simulink model "VerificaLQR"  (R2025b)
settings: Solver=VariableStepAuto  StartTime=0.0  StopTime=10.0  RelTol=1e-3
values from neighbouring files (symbols this model uses):
  r = 129    [matrci_ridotte.mat]
undefined symbols (not defined in the file or in its folder): A, B, C_LQR, D, K_LQR_i, K_LQR_x
settings Model: Creator=salvo  LastModifiedBy=salvo

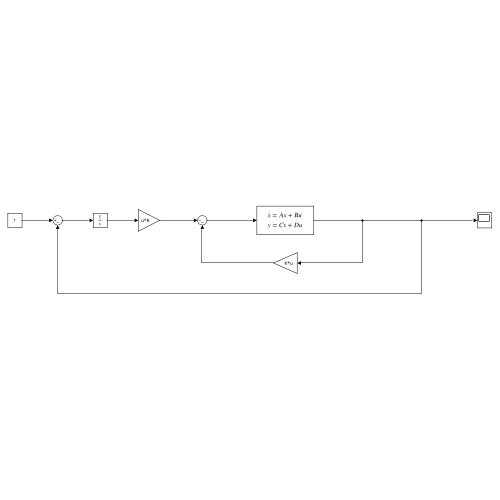
[thumbnail: Simulink's stored preview of the top-level diagram]
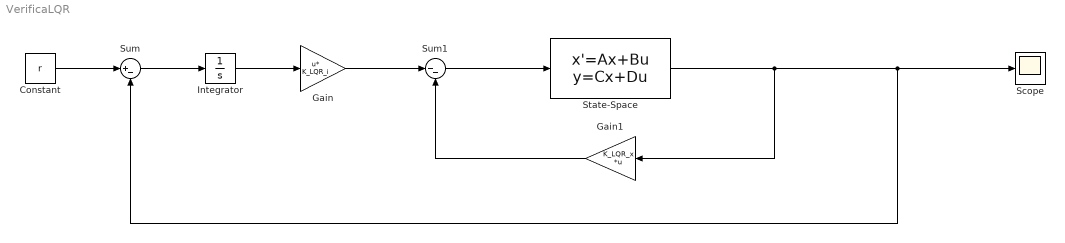
== system VerificaLQR ==
  Constant : Constant  Value=r
  Gain : Gain  Gain=K_LQR_i  Multiplication=Matrix(u*K)
  Gain1 : Gain  Gain=K_LQR_x  Multiplication=Matrix(K*u)
  Integrator : Integrator
  Scope : Scope
      settings: ActiveDisplayYMinimum=-215.38255837589762  ActiveDisplayYMaximum=283.465522017225
  State-Space : StateSpace  A=A  B=B  C=C_LQR  D=D  InitialCondition=0
  Sum : Sum  Inputs=|+-
  Sum1 : Sum  Inputs=|--
  wires:
  Gain1/1 -> Sum1/2
  Constant/1 -> Sum/1
  Integrator/1 -> Gain/1
  Sum1/1 -> State-Space/1
  Gain/1 -> Sum1/1
  State-Space/1 -> Gain1/1, Sum/2, Scope/1
  Sum/1 -> Integrator/1
